simulink subsystem "Circuit_CT_SS_Noise"  (R2022a)
settings: Solver=VariableStepAuto  StartTime=0.0  StopTime=10.0  RelTol=1e-3
values from neighbouring files (symbols this model uses):
  C = [1 0 ... (first row only)    [TestDiscreteTimeSimulink.m]
  Q = Q_0*eye(N_inputs)    [TestDiscreteTimeSimulink.m]
  R = R_0*eye(N_meas)    [TestDiscreteTimeSimulink.m]
undefined symbols (not defined in the file or in its folder): A_CT, B_CT, x0
settings Model: Creator=tyevans  LastModifiedBy=tyevans

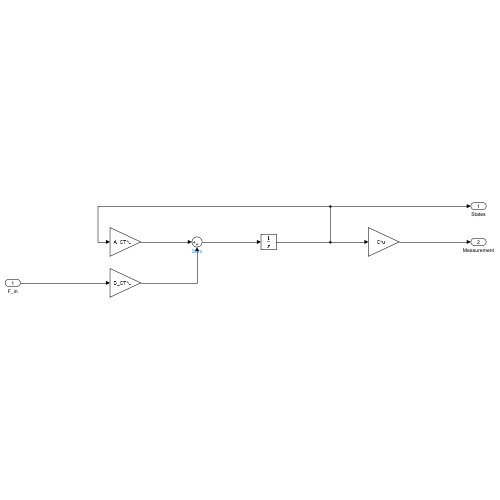
[thumbnail: Simulink's stored preview of the top-level diagram]
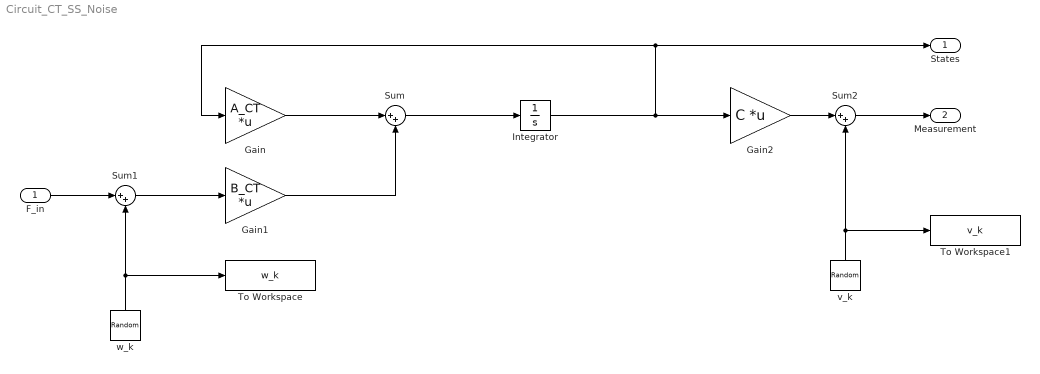
== system Circuit_CT_SS_Noise ==
  F_in : Inport
  Gain : Gain  Gain=A_CT  Multiplication=Matrix(K*u)
  Gain1 : Gain  Gain=B_CT  Multiplication=Matrix(K*u)
  Gain2 : Gain  Gain=C  Multiplication=Matrix(K*u)
  Integrator : Integrator  InitialCondition=x0
  Sum : Sum  Inputs=|++
  Sum1 : Sum  Inputs=|++
  Sum2 : Sum  Inputs=|++
  To Workspace : ToWorkspace  VariableName=w_k  SaveFormat=Structure With Time  SampleTime=-1
  To Workspace1 : ToWorkspace  VariableName=v_k  SaveFormat=Structure With Time  SampleTime=-1
  v_k : RandomNumber  Variance=R  Seed=1  SampleTime=1  VectorParams1D=off
  w_k : RandomNumber  Variance=Q  Seed=1  SampleTime=1  VectorParams1D=off
  States : Outport
  Measurement : Outport  Port=2
  wires:
  Integrator/1 -> Gain2/1, Gain/1, States/1
  Gain/1 -> Sum/1
  Sum/1 -> Integrator/1
  Gain1/1 -> Sum/2
  Sum1/1 -> Gain1/1
  F_in/1 -> Sum1/1
  w_k/1 -> To Workspace/1, Sum1/2
  v_k/1 -> To Workspace1/1, Sum2/2
  Gain2/1 -> Sum2/1
  Sum2/1 -> Measurement/1
